simulink model "adaptation_part2"  (R2023a)
settings: Solver=ode3  StartTime=0.0  StopTime=8  FixedStep=0.001  RelTol=1e-3
values from neighbouring files (symbols this model uses):
  beta1 = optsect(1)    [adaptation_sim_part1.m]    (also in adaptation_sim_part2.m; evaluations.m = sectors(i,1); evaluations.mat = [0 0.4 0.8]; nonlinearities.mat = [0 0.4 0.8])
  beta2 = optsect(3)    [adaptation_sim_part1.m]    (also in adaptation_sim_part2.m; evaluations.m = sectors(i,3); evaluations.mat = [0 0.5 1]; nonlinearities.mat = [0 0.5 1])
  betak1 = optsect(2)    [adaptation_sim_part1.m]    (also in adaptation_sim_part2.m; s_ts22.m)
  betak2 = optsect(4)    [adaptation_sim_part1.m]    (also in adaptation_sim_part2.m; s_ts22.m)
  bp1 = NL1opt.BreakPoints    [adaptation_sim_part1.m]    (also in adaptation_sim_part2.m; refmodel.m = NL1{i}.BreakPoints)
  bp2 = NL2opt.BreakPoints    [adaptation_sim_part1.m]    (also in adaptation_sim_part2.m; refmodel.m = NL2{j}.BreakPoints)
  H = [1  1  0; 0.5  0  1]    [evaluations.mat]    (also in nonlinearities.mat; project.m = [  1,1,0)
  M1 = bp1(1,:)    [adaptation_sim_part1.m]    (also in adaptation_sim_part2.m; s_ts22.m)
  M2 = bp2(1,:)    [adaptation_sim_part1.m]    (also in adaptation_sim_part2.m; s_ts22.m)
  x0 = [1,1,1]    [adaptation_sim_part1.m]    (also in adaptation_sim_part2.m = [1,-1,1]; evaluations.m = [x01(a),x02(b),x03(c)]'; refmodel.m = [1,0,-0.6]; s_ts22.m = [])
settings Model: Creator=kwiktor  LastModifiedBy=kwiktor
settings DebuggingCC: UnconnectedInputMsg=warning  UnconnectedOutputMsg=warning  UnconnectedLineMsg=warning
settings ModelReferenceCC: EnableRefExpFcnMdlSchedulingChecks=on
settings SFSimCC: SimTargetLang=C++  GPUAcceleration=on  SimDLTargetLibrary=cudnn
settings RTWCC: DLArmComputeVersion=19.05

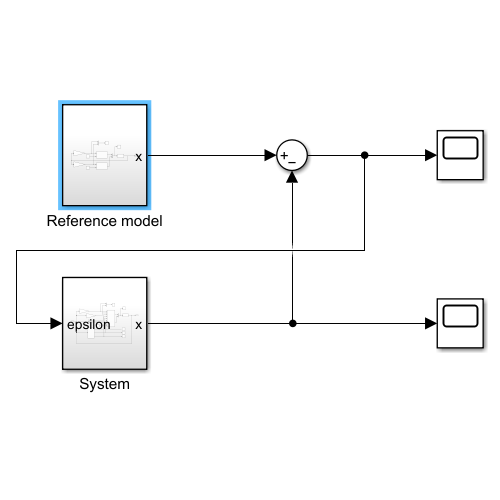
[thumbnail: Simulink's stored preview of the top-level diagram]
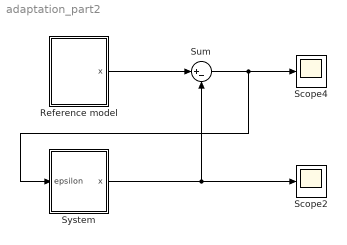
== system adaptation_part2 ==
  Reference model : Subsystem
  Scope2 : Scope
  Scope4 : Scope
  Sum : Sum  Inputs=|+-
  System : Subsystem
  wires:
  Reference model/1(x) -> Sum/1
  Sum/1 -> System/1(epsilon), Scope4/1
  System/1(x) -> Sum/2, Scope2/1

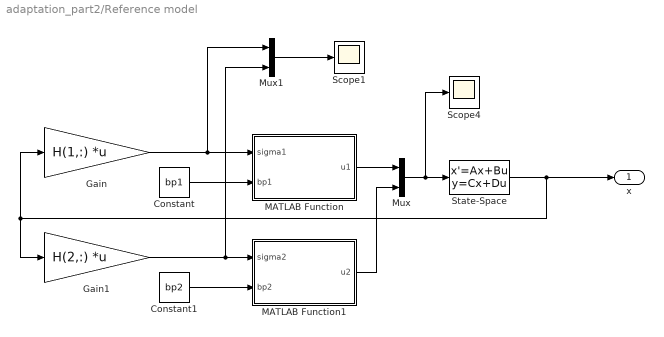
== system adaptation_part2/Reference model ==
  Constant : Constant  Value=bp1
  Constant1 : Constant  Value=bp2
  Gain : Gain  Gain=H(1,:)  Multiplication=Matrix(K*u)
  Gain1 : Gain  Gain=H(2,:)  Multiplication=Matrix(K*u)
  MATLAB Function : MATLAB Function  TreatAsAtomicUnit=on
  MATLAB Function1 : MATLAB Function  TreatAsAtomicUnit=on
  Mux : Mux  Inputs=2
  Mux1 : Mux  Inputs=2
  Scope1 : Scope
  Scope4 : Scope
  State-Space : StateSpace  A=[-4,-9,-10; 1,0,0; 0,1,0]  B=[2,-1; 0,1; 1,0]  C=eye(3)  D=zeros(3,2)  InitialCondition=x0
  x : Outport
  wires:
  Mux/1 -> Scope4/1, State-Space/1
  State-Space/1 -> x/1, Gain/1, Gain1/1
  Gain/1 -> Mux1/1, MATLAB Function/1(sigma1)
  Gain1/1 -> Mux1/2, MATLAB Function1/1(sigma2)
  MATLAB Function/1(u1) -> Mux/1
  Constant1/1 -> MATLAB Function1/2(bp2)
  MATLAB Function1/1(u2) -> Mux/2
  Mux1/1 -> Scope1/1
  Constant/1 -> MATLAB Function/2(bp1)

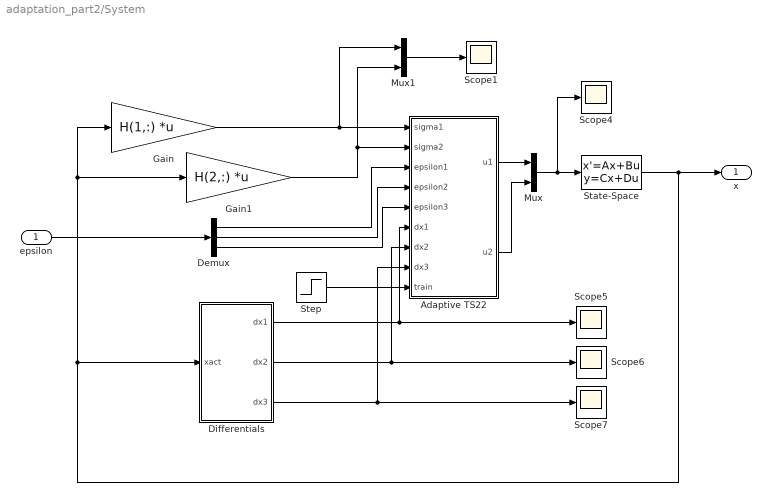
== system adaptation_part2/System ==
  epsilon : Inport
  Adaptive TS22 : Subsystem  mask{M1=M1, M2=M2, beta1=beta1, betak1=betak1, beta2=beta2, betak2=betak2}
      mask prompts: M1 "Wierzcholki zbiorow dla x1:"; M2 "Wierzcholki zbiorow dla x2:"; betak1 "beta1 + k1:"; betak2 "beta2 + k2:"
  Demux : Demux  Outputs=3
  Differentials : Subsystem
  Gain : Gain  Gain=H(1,:)  Multiplication=Matrix(K*u)
  Gain1 : Gain  Gain=H(2,:)  Multiplication=Matrix(K*u)
  Mux : Mux  Inputs=2
  Mux1 : Mux  Inputs=2
  Scope{1,4..7} (5 alike) : Scope
  State-Space : StateSpace  A=[-4,-9,-10; 1,0,0; 0,1,0]  B=[2,-1; 0,1; 1,0]  C=eye(3)  D=zeros(3,2)  InitialCondition=x0
  Step : Step  Time=0  SampleTime=0
  x : Outport
  wires:
  Mux/1 -> Scope4/1, State-Space/1
  State-Space/1 -> x/1, Gain/1, Gain1/1, Differentials/1(xact)
  Gain/1 -> Mux1/1, Adaptive TS22/1(sigma1)
  Adaptive TS22/1(u1) -> Mux/1
  Adaptive TS22/2(u2) -> Mux/2
  Mux1/1 -> Scope1/1
  Gain1/1 -> Mux1/2, Adaptive TS22/2(sigma2)
  epsilon/1 -> Demux/1
  Demux/1 -> Adaptive TS22/3(epsilon1)
  Demux/2 -> Adaptive TS22/4(epsilon2)
  Demux/3 -> Adaptive TS22/5(epsilon3)
  Differentials/2(dx2) -> Scope6/1, Adaptive TS22/7(dx2)
  Differentials/3(dx3) -> Scope7/1, Adaptive TS22/8(dx3)
  Differentials/1(dx1) -> Scope5/1, Adaptive TS22/6(dx1)
  Step/1 -> Adaptive TS22/9(train)

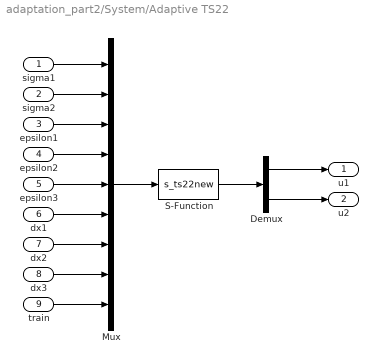
== system adaptation_part2/System/Adaptive TS22 ==
  sigma1 : Inport
  sigma2 : Inport  Port=2
  epsilon1 : Inport  Port=3
  epsilon2 : Inport  Port=4
  epsilon3 : Inport  Port=5
  dx1 : Inport  Port=6
  dx2 : Inport  Port=7
  dx3 : Inport  Port=8
  train : Inport  Port=9
  Demux : Demux  Outputs=2
  Mux : Mux  Inputs=9
  S-Function : S-Function  FunctionName=s_ts22new  Parameters=M1,M2,beta1,betak1,beta2,betak2  SFunctionDeploymentMode=off  EnableBusSupport=off
  u1 : Outport
  u2 : Outport  Port=2
  wires:
  Demux/2 -> u2/1
  Demux/1 -> u1/1
  Mux/1 -> S-Function/1
  sigma1/1 -> Mux/1
  sigma2/1 -> Mux/2
  epsilon1/1 -> Mux/3
  epsilon3/1 -> Mux/5
  epsilon2/1 -> Mux/4
  dx1/1 -> Mux/6
  dx2/1 -> Mux/7
  train/1 -> Mux/9
  dx3/1 -> Mux/8
  S-Function/1 -> Demux/1

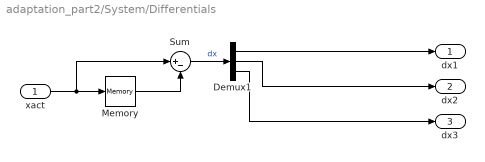
== system adaptation_part2/System/Differentials ==
  xact : Inport
  Demux1 : Demux  Outputs=3
  Memory : Memory
  Sum : Sum  Inputs=|+-
  dx1 : Outport
  dx2 : Outport  Port=2
  dx3 : Outport  Port=3
  wires:
  Demux1/3 -> dx3/1
  Demux1/1 -> dx1/1
  xact/1 -> Sum/1, Memory/1
  Memory/1 -> Sum/2
  Sum/1 -> Demux1/1  "dx"
  Demux1/2 -> dx2/1

== matlab function adaptation_part2/Reference model/MATLAB Function ==
  data: sigma1 input; u1 output; bp1 input
function u1 = fcn1(sigma1, bp1)

% linear controller
%u1 = bp1*sigma1;

% nonlinear controller
u1 = evaluatenl(bp1,sigma1);

== matlab function adaptation_part2/Reference model/MATLAB Function1 ==
  data: sigma2 input; u2 output; bp2 input
function u2 = fcn2(sigma2, bp2)

% regulator liniowy
%u2 = bp2*sigma2;

% regulator nieliniowy
u2 = evaluatenl(bp2,sigma2);
